simulink model "lightcontrol"  (R2020a)
settings: Solver=VariableStepAuto  StartTime=0.0  StopTime=10.0  RelTol=1e-3
libraries: arduinolib x6
settings Model: Creator=pc  LastModifiedBy=pc

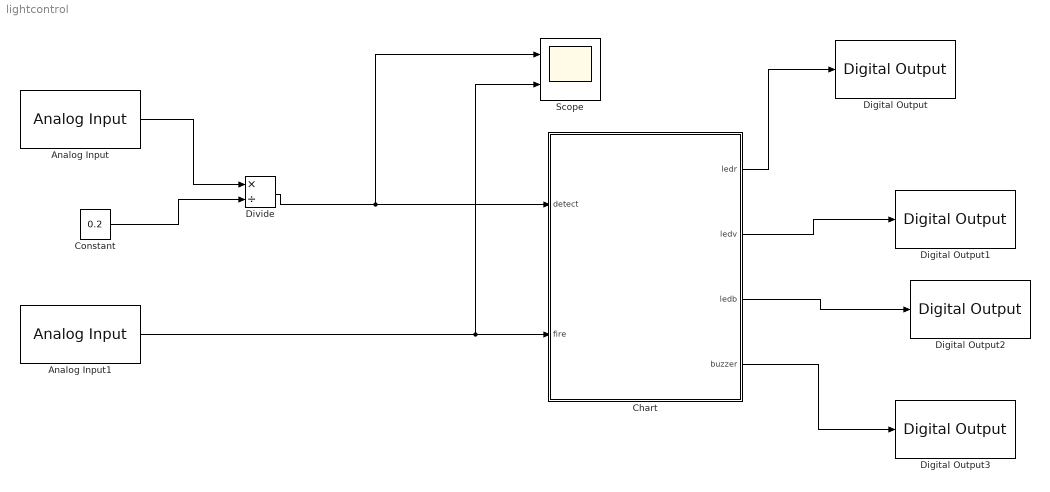
== system lightcontrol ==
  Analog Input : arduinolib/Analog Input  pinNumber=4  ReadResultsOnly=off  ConversionTriggerSource=Software  ExternalTriggerType=uint32( 0 )  OutputDataType=uint16  EnableConversionCompleteNotify=off  EnableOuputStatus=off  SampleTime=-1  blockPlatform=arduino
  Analog Input1 : arduinolib/Analog Input  pinNumber=4  ReadResultsOnly=off  ConversionTriggerSource=Software  ExternalTriggerType=uint32( 0 )  OutputDataType=uint16  EnableConversionCompleteNotify=off  EnableOuputStatus=off  SampleTime=-1  blockPlatform=arduino
  Chart : Stateflow chart  TreatAsAtomicUnit=on
  Constant : Constant  Value=0.2
  Digital Output : arduinolib/Digital Output  pinNumber=9  Direction=output  blockPlatform=arduino
  Digital Output1 : arduinolib/Digital Output  pinNumber=8  Direction=output  blockPlatform=arduino
  Digital Output2 : arduinolib/Digital Output  pinNumber=7  Direction=output  blockPlatform=arduino
  Digital Output3 : arduinolib/Digital Output  pinNumber=5  Direction=output  blockPlatform=arduino
  Divide : Product  Inputs=*/
  Scope : Scope  NumInputPorts=2
  wires:
  Chart/1(ledr) -> Digital Output/1
  Chart/2(ledv) -> Digital Output1/1
  Chart/3(ledb) -> Digital Output2/1
  Chart/4(buzzer) -> Digital Output3/1
  Analog Input1/1 -> Chart/2(fire), Scope/2
  Divide/1 -> Scope/1, Chart/1(detect)
  Analog Input/1 -> Divide/1
  Constant/1 -> Divide/2

== stateflow chart lightcontrol/Chart ==
  state LEDR
    ledr=1;
    buzzer=0;
  state LEDV
    ledv=1;
    buzzer=1;
  state LEDB
    ledb=1;
    buzzer=0;
  (default) -> LEDR
  LEDR -> LEDV : [detect <=400]
  LEDB -> LEDR : [detect >400 && fire>50]
  LEDV -> LEDB : [fire<=50]
  data: ledr output; ledv output; ledb output; buzzer output; detect input; fire input
